simulink model "file_1"  (R2022a)
settings: Solver=FixedStepDiscrete  StartTime=0.0  StopTime=inf  RelTol=1e-3
libraries: androidcommunicationlib x6, androidaudiovideolib x1, androidsensorlib x1
settings Model: Creator=GautamVashishtha  LastModifiedBy=GautamVashishtha
settings OptimizationCC: EnhancedBackFolding=on  PassReuseOutputArgsAs=Individual arguments  ZeroExternalMemoryAtStartup=off  ZeroInternalMemoryAtStartup=off  MaxStackSize=64  OptimizeBlockOrder=speed  DifferentSizesBufferReuse=on  OptimizationCustomize=off  EfficientTunableParamExpr=on
settings DebuggingCC: ParameterTunabilityLossMsg=error
settings HardwareCC: ProdBitPerPointer=32  ProdBitPerSizeT=32  ProdBitPerPtrDiffT=32  ProdLargestAtomicInteger=Long  ProdLargestAtomicFloat=Double  ProdWordSize=32  ProdHWDeviceType=ARM Compatible->ARM Cortex  UseEmbeddedCoderFeatures=off  UseSimulinkCoderFeatures=off
settings SFSimCC: MATLABDynamicMemAlloc=off
settings RTWCC: SystemTargetFile=ert.tlc  HardwareBoard=Android Device  TLCOptions="-aInlineSetEventsForThisBaseRateFcn=TLC_FALSE -aSuppressMultiTaskScheduler=TLC_FALSE  -aRateBasedStepFcn=0"  TemplateMakefile=ert_default_tmf  RTWVerbose=off  Toolchain=Android SDK/NDK Tools
settings CodeAppCC: ForceParamTrailComments=on  IgnoreCustomStorageClasses=off  OperatorAnnotations=on  SimulinkDataObjDesc=on  SFDataObjDesc=on  InsertBlockDesc=on
settings ERTTargetCC: SupportNonInlinedSFcns=on

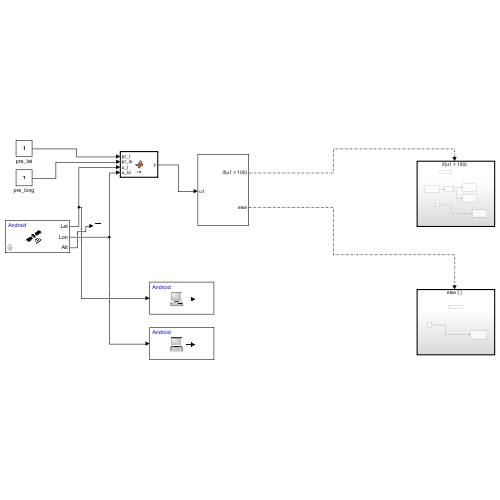
[thumbnail: Simulink's stored preview of the top-level diagram]
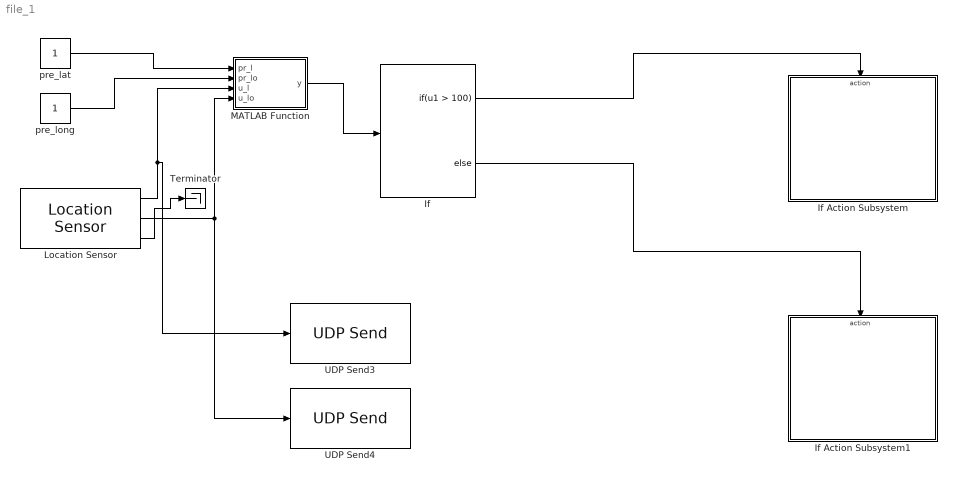
== system file_1 ==
  If : If  IfExpression=u1 > 100
  If Action Subsystem : Subsystem  TreatAsAtomicUnit=on
  If Action Subsystem1 : Subsystem  TreatAsAtomicUnit=on
  Location Sensor : androidsensorlib/Location Sensor  OutputVector=off  SampleTime=0.1  BlockPlatform=Android
      settings: SourceProductBaseCode=ANDROID
  MATLAB Function : MATLAB Function  TreatAsAtomicUnit=on
  Terminator : Terminator
  UDP Send3 : androidcommunicationlib/UDP Send  remoteURL='10.7.57.20'  remotePort=5000  localURL='0.0.0.0'  localPortSource=Automatically determine  localPort=-1  sampletime=-1  blockPlatform=Android  separateLengthPort=0
      settings: SourceProductBaseCode=ANDROID
  UDP Send4 : androidcommunicationlib/UDP Send  remoteURL='10.7.57.20'  remotePort=4000  localURL='0.0.0.0'  localPortSource=Automatically determine  localPort=-1  sampletime=-1  blockPlatform=Android  separateLengthPort=0
      settings: SourceProductBaseCode=ANDROID
  pre_lat : Constant
  pre_long : Constant
  wires:
  Location Sensor/1 -> UDP Send3/1, MATLAB Function/3(u_l)
  Location Sensor/2 -> UDP Send4/1, MATLAB Function/4(u_lo)
  Location Sensor/3 -> Terminator/1
  pre_lat/1 -> MATLAB Function/1(pr_l)
  pre_long/1 -> MATLAB Function/2(pr_lo)
  MATLAB Function/1(y) -> If/1
  If/1 -> If Action Subsystem/Action
  If/2 -> If Action Subsystem1/Action

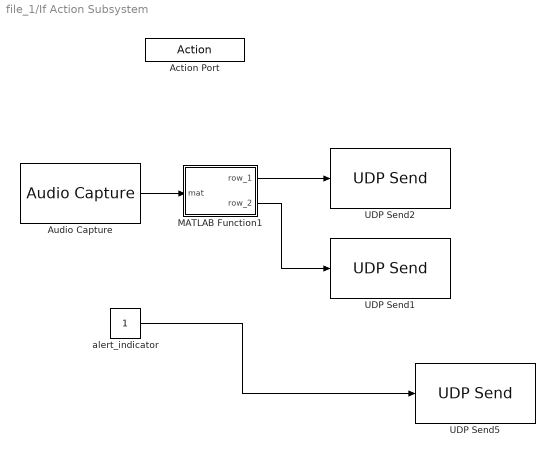
== system file_1/If Action Subsystem ==
  Action Port : ActionPort  ActionPortLabel=if(u1 > 100)
  Audio Capture : androidaudiovideolib/Audio Capture  SampleFreq=44100  FrameSize=4410  SampleTime=0.1  SimulateUsing=Code generation  DeviceStr=0  QueueDuration=0  BlockPlatform=Android  AudioSamplingFreq=44100
      settings: SourceProductBaseCode=ANDROID
  MATLAB Function1 : MATLAB Function  TreatAsAtomicUnit=on
  UDP Send1 : androidcommunicationlib/UDP Send  remoteURL='10.7.57.20'  remotePort=8000  localURL='0.0.0.0'  localPortSource=Automatically determine  localPort=-1  sampletime=-1  blockPlatform=Android  separateLengthPort=0
      settings: SourceProductBaseCode=ANDROID
  UDP Send2 : androidcommunicationlib/UDP Send  remoteURL='10.7.57.20'  remotePort=6000  localURL='0.0.0.0'  localPortSource=Automatically determine  localPort=-1  sampletime=-1  blockPlatform=Android  separateLengthPort=0
      settings: SourceProductBaseCode=ANDROID
  UDP Send5 : androidcommunicationlib/UDP Send  remoteURL='10.7.57.20'  remotePort=3000  localURL='0.0.0.0'  localPortSource=Automatically determine  localPort=-1  sampletime=-1  blockPlatform=Android  separateLengthPort=0
      settings: SourceProductBaseCode=ANDROID
  alert_indicator : Constant
  wires:
  MATLAB Function1/2(row_2) -> UDP Send1/1
  MATLAB Function1/1(row_1) -> UDP Send2/1
  Audio Capture/1 -> MATLAB Function1/1(mat)
  alert_indicator/1 -> UDP Send5/1

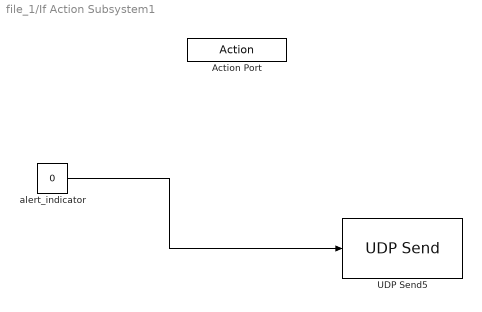
== system file_1/If Action Subsystem1 ==
  Action Port : ActionPort  ActionPortLabel=else
  UDP Send5 : androidcommunicationlib/UDP Send  remoteURL='10.7.57.20'  remotePort=3000  localURL='0.0.0.0'  localPortSource=Automatically determine  localPort=-1  sampletime=-1  blockPlatform=Android  separateLengthPort=0
      settings: SourceProductBaseCode=ANDROID
  alert_indicator : Constant  Value=0
  wires:
  alert_indicator/1 -> UDP Send5/1

== matlab function file_1/If Action Subsystem/MATLAB Function1 ==
  data: mat input; row_1 output; row_2 output
function [row_1,row_2] = fcn(mat)
row_1_ = mat(1,:);
row_2_ = mat(2,:);
row_1 = row_1_;
row_2 = row_2_;

== matlab function file_1/MATLAB Function ==
  data: pr_l input; y output; pr_lo input; u_l input; u_lo input
function y = fcn(pr_l,pr_lo,u_l,u_lo)
R = 6371;                      
delta_lat = pr_l  - u_l;
delta_lon = pr_lo - u_lo;    
a = sin(delta_lat/2)^2 + cos(pr_lo) * cos(u_lo) * ...
    sin(delta_lon/2)^2;
c = 2 * atan2(sqrt(a), sqrt(1-a));
km = R * c;
y = km*1000;
